simulink model "SF015A_WhlImbRejctn"  (R2013b)
settings: Solver=FixedStepDiscrete  SolverMode=SingleTasking  StartTime=0.0  StopTime=1  FixedStep=0.002  RelTol=1e-3
undefined symbols (not defined in the file): ACTIVBANDMAX_ULS_U32, ADAPVFILMAX_ULS_F32, ADJOUTPMAX_ULS_F32, ARCHGLBPRM_180OVERPI_ULS_F32, ARCHGLBPRM_2MILLISEC_SEC_F32, ARCHGLBPRM_2PI_ULS_F32, ARCHGLBPRM_FLOATZEROTHD_ULS_F32, ARCHGLBPRM_PI_ULS_F32, ARCHGLBPRM_PIOVER180_ULS_F32, ARCHGLBPRM_PIOVER2_ULS_F32, CALMINSPERCOUNT_ULS_F32, Cntr, DURATIONDISABLE_CNT_U16, FILTWHLSPDMAX_MOTRADPERSEC_F32, FRQMIN_ULS_F32, MICROSECTOMILLISEC_ULS_F32, MINSTOMILLISEC_ULS_F32, NINETY_ULS_F32, NODEBSTEP_CNT_U16, NROFDLY_CNT_U08, NtcSts1, NvmGetErrSts1, ONEHALF_ULS_F32, ONEHUNDRED_ULS_F32, ONEOVRTHREE_ULS_F32, ONEOVRTWENTY_ULS_F32, ONETHOUSAND_ULS_F32, PEAKMAX_ULS_F32, PEAKMIN_ULS_F32, PHAADJMAX_ULS_F32, PITIMESSAMPLETIME_ULS_F32, SigQlfr1, STOREDMINSPERCOUNT_ULS_F32, Sts, SysSt1, TWO_ULS_F32, TWOOVRTHREE_ULS_F32, UGRFILMAX_ULS_F32, WhlImbRejctnAdpvFac, WhlImbRejctnAutScaEna, WhlImbRejctnAutScaTar, WhlImbRejctnCurrMgnSlewPerLoop, WhlImbRejctnDcTrendFltRcvryDly, WhlImbRejctnDcTrendFltRcvryNegStep, WhlImbRejctnDcTrendFltRcvryPosStep, WhlImbRejctnDcTrendFltRcvryThd, WhlImbRejctnDcTrendTh2Tq, WhlImbRejctnDcTrendThTq, WhlImbRejctnDcTrendTi2Sec, WhlImbRejctnDcTrendTiSec, WhlImbRejctnEnaSlewPerLoop, WhlImbRejctnFctEna, WhlImbRejctnFltNtc, WhlImbRejctnFrqDiagcAmpThd, WhlImbRejctnFrqDiagcEna, WhlImbRejctnFrqDiagcFltRcvryDly, WhlImbRejctnFrqDiagcFltRcvryNegStep, WhlImbRejctnFrqDiagcFltRcvryPosStep, WhlImbRejctnFrqDiagcFltRcvryThd, WhlImbRejctnFrqDiagcThd ... (+30)
libraries: FixdToFloat x32, simulink x26, NxtrLim x25, Fil x20, NxtrAbslt x9, NxtrMath x7, NxtrMax x6, NxtrMin x4, NxtrNvM x2, FloatToFixd x2, LnrIntrpn x2, NxtrSign x1
(part 9 of 14)

== system SF015A_WhlImbRejctn/WhlImbRejctn/WhlImbRejctnPer2/WIR Low Speed Diagnostics/MaxPersisDiag/If Action Subsystem ==
  In1 : Inport
  Action Port : ActionPort  ActionType=then
  CopyRight2 : Subsystem  Description=|  mask(Copyright Information){none=on}
      | Copyright info block.                                               
      |                                                                     
      | Place copyright information at the top of every subsystem in design.
      mask prompts: none "No parameters"
      mask help: Place copyright information at the top of every subsystem in design.
      mask Display:
      | NxtrConf = 'Nexteer Confidential';
      | 
      | sys = bdroot; %handle for the current model ("system")
      | first = get_param(sys,'Created');
      | if(isempty(first))
      |     first = datestr(now,'yyyy');
      | else
      |     first = first(end-3:end);  %year is last four digits
      | end
      | 
      | last = get_param(sys,'LastModifiedDate');
      | if isempty(last)
      |     last = datestr(now,'yyyy');
      | else
      |     last = last(end-3:end);
      | end
      | 
      | if strcmp(first,last)
      |     fprintf('%s -- Copyright %s Nexteer',NxtrConf,first)
      | else
      |     fprintf('%s -- %s%s- %s Nexteer',NxtrConf,char(169),first,last)
      | end
  Out1 : Outport
  wires:
  In1/1 -> Out1/1

== system SF015A_WhlImbRejctn/WhlImbRejctn/WhlImbRejctnPer2/WIR Low Speed Diagnostics/MaxPersisDiag/Update Persistence Band 3 ==
  NVM Var : Inport
  Condition : Inport  Port=2
  Add : Sum
  Constant3 : Constant  OutDataTypeStr=uint32
  Constant6 : Constant  RequirementInfo={} %GIDa_1d525a57_12aa_4786_b039_fdbfeffc8f33  Value=ACTIVBANDMAX_ULS_U32
  CopyRight2 : Subsystem  Description=|  mask(Copyright Information){none=on}
      | Copyright info block.                                               
      |                                                                     
      | Place copyright information at the top of every subsystem in design.
      mask prompts: none "No parameters"
      mask help: Place copyright information at the top of every subsystem in design.
      mask Display:
      | NxtrConf = 'Nexteer Confidential';
      | 
      | sys = bdroot; %handle for the current model ("system")
      | first = get_param(sys,'Created');
      | first = first(end-3:end);  %year is last four digits
      | 
      | last = get_param(sys,'LastModifiedDate');
      | if isempty(last)
      |     last = datestr(now,'yyyy');
      | else
      |     last = last(end-3:end);
      | end
      | 
      | if strcmp(first,last)
      |     fprintf('%s -- Copyright %s Nexteer',NxtrConf,first)
      | else
      |     fprintf('%s -- %s%s- %s Nexteer',NxtrConf,char(169),first,last)
      | end
  FreqDiagFault1 : Subsystem  RequirementInfo={} %GIDa_be7adfbe_12e3_4d1f_b751_a499999159a7  TreatAsAtomicUnit=on
  If1 : If  RequirementInfo={} %GIDa_0ea92c53_6d11_40e6_981f_8602e62ea0c9  IfExpression=u1
  Logical Operator1 : Logic  AllPortsSameDT=off  OutDataTypeStr=boolean
  Merge1 : Merge
  NoFault1 : Subsystem  RequirementInfo={} %GIDa_03ebdbb3_7e71_4f28_811c_205b7f9dc526  TreatAsAtomicUnit=on
  Relational Operator7 : RelationalOperator  RequirementInfo={} %GIDa_01722b6f_ba93_4b03_83b3_204efa7b0808  Operator=<  OutDataTypeStr=boolean
  UpdateVar : Outport
  wires:
  Logical Operator1/1 -> If1/1
  FreqDiagFault1/1(Output) -> Merge1/1
  NoFault1/1(Output) -> Merge1/2
  If1/1 -> FreqDiagFault1/Action
  If1/2 -> NoFault1/Action
  Constant3/1 -> Add/1
  Add/1 -> FreqDiagFault1/1(Input)
  NVM Var/1 -> [Var]
  Condition/1 -> Logical Operator1/1
  Constant6/1 -> Relational Operator7/2
  Relational Operator7/1 -> Logical Operator1/2
  [Var] -> Relational Operator7/1
  [Var] -> Add/2
  [Var] -> NoFault1/1(Input)
  Merge1/1 -> UpdateVar/1

== system SF015A_WhlImbRejctn/WhlImbRejctn/WhlImbRejctnPer2/WIR Low Speed Diagnostics/MaxPersisDiag/Update Persistence Band1 ==
  NVM Var : Inport
  Condition : Inport  Port=2
  Add : Sum
  Constant3 : Constant  OutDataTypeStr=uint32
  Constant6 : Constant  RequirementInfo={} %GIDa_d3879db0_aaaa_4f96_8253_c1a666713adb  Value=ACTIVBANDMAX_ULS_U32
  CopyRight2 : Subsystem  Description=|  mask(Copyright Information){none=on}
      | Copyright info block.                                               
      |                                                                     
      | Place copyright information at the top of every subsystem in design.
      mask prompts: none "No parameters"
      mask help: Place copyright information at the top of every subsystem in design.
      mask Display:
      | NxtrConf = 'Nexteer Confidential';
      | 
      | sys = bdroot; %handle for the current model ("system")
      | first = get_param(sys,'Created');
      | first = first(end-3:end);  %year is last four digits
      | 
      | last = get_param(sys,'LastModifiedDate');
      | if isempty(last)
      |     last = datestr(now,'yyyy');
      | else
      |     last = last(end-3:end);
      | end
      | 
      | if strcmp(first,last)
      |     fprintf('%s -- Copyright %s Nexteer',NxtrConf,first)
      | else
      |     fprintf('%s -- %s%s- %s Nexteer',NxtrConf,char(169),first,last)
      | end
  FreqDiagFault1 : Subsystem  RequirementInfo={} %GIDa_359f150f_d6cc_4ff0_a268_6ba457e2d369  TreatAsAtomicUnit=on
  If1 : If  RequirementInfo={} %GIDa_06089e48_f5cb_45cb_89f4_21bbb0bce6ae  IfExpression=u1
  Logical Operator1 : Logic  AllPortsSameDT=off  OutDataTypeStr=boolean
  Merge1 : Merge
  NoFault1 : Subsystem  RequirementInfo={} %GIDa_63cd9bcc_abfd_4796_b9a9_88c94dc82f42  TreatAsAtomicUnit=on
  Relational Operator7 : RelationalOperator  RequirementInfo={} %GIDa_95dc9f26_2408_4902_80b2_c9582cdf1274  Operator=<  OutDataTypeStr=boolean
  UpdateVar : Outport
  wires:
  Logical Operator1/1 -> If1/1
  FreqDiagFault1/1(Output) -> Merge1/1
  NoFault1/1(Output) -> Merge1/2
  If1/1 -> FreqDiagFault1/Action
  If1/2 -> NoFault1/Action
  Constant3/1 -> Add/1
  Add/1 -> FreqDiagFault1/1(Input)
  NVM Var/1 -> [Var]
  Condition/1 -> Logical Operator1/1
  Constant6/1 -> Relational Operator7/2
  Relational Operator7/1 -> Logical Operator1/2
  [Var] -> Relational Operator7/1
  [Var] -> NoFault1/1(Input)
  [Var] -> Add/2
  Merge1/1 -> UpdateVar/1

== system SF015A_WhlImbRejctn/WhlImbRejctn/WhlImbRejctnPer2/WIR Low Speed Diagnostics/MaxPersisDiag/Update Persistence Band2 ==
  NVM Var : Inport
  Condition : Inport  Port=2
  Add : Sum
  Constant3 : Constant  OutDataTypeStr=uint32
  Constant6 : Constant  RequirementInfo={} %GIDa_82db90a7_98d3_4902_8915_0b7af750842f  Value=ACTIVBANDMAX_ULS_U32
  CopyRight2 : Subsystem  Description=|  mask(Copyright Information){none=on}
      | Copyright info block.                                               
      |                                                                     
      | Place copyright information at the top of every subsystem in design.
      mask prompts: none "No parameters"
      mask help: Place copyright information at the top of every subsystem in design.
      mask Display:
      | NxtrConf = 'Nexteer Confidential';
      | 
      | sys = bdroot; %handle for the current model ("system")
      | first = get_param(sys,'Created');
      | first = first(end-3:end);  %year is last four digits
      | 
      | last = get_param(sys,'LastModifiedDate');
      | if isempty(last)
      |     last = datestr(now,'yyyy');
      | else
      |     last = last(end-3:end);
      | end
      | 
      | if strcmp(first,last)
      |     fprintf('%s -- Copyright %s Nexteer',NxtrConf,first)
      | else
      |     fprintf('%s -- %s%s- %s Nexteer',NxtrConf,char(169),first,last)
      | end
  FreqDiagFault1 : Subsystem  RequirementInfo={} %GIDa_6ea3fd2e_fad0_4c9e_828f_0553c62f3183  TreatAsAtomicUnit=on
  If1 : If  RequirementInfo={} %GIDa_3d6838fe_19df_4745_9894_1f41b327ce7a  IfExpression=u1
  Logical Operator1 : Logic  AllPortsSameDT=off  OutDataTypeStr=boolean
  Merge1 : Merge
  NoFault1 : Subsystem  RequirementInfo={} %GIDa_4a4caa65_5361_47b0_a88d_ff799b187767  TreatAsAtomicUnit=on
  Relational Operator7 : RelationalOperator  RequirementInfo={} %GIDa_673935b7_bbed_4a45_bb15_19f10e0d5d6b  Operator=<  OutDataTypeStr=boolean
  UpdateVar : Outport
  wires:
  Logical Operator1/1 -> If1/1
  FreqDiagFault1/1(Output) -> Merge1/1
  NoFault1/1(Output) -> Merge1/2
  If1/1 -> FreqDiagFault1/Action
  If1/2 -> NoFault1/Action
  Constant3/1 -> Add/1
  Add/1 -> FreqDiagFault1/1(Input)
  NVM Var/1 -> [Var]
  Condition/1 -> Logical Operator1/1
  [Var] -> Relational Operator7/1
  Constant6/1 -> Relational Operator7/2
  Relational Operator7/1 -> Logical Operator1/2
  [Var] -> Add/2
  [Var] -> NoFault1/1(Input)
  Merge1/1 -> UpdateVar/1

== system SF015A_WhlImbRejctn/WhlImbRejctn/WhlImbRejctnInit1/Check NVM Data/CheckCompPersistence/NoFault/CopyRight2 ==

== system SF015A_WhlImbRejctn/WhlImbRejctn/WhlImbRejctnInit1/Check NVM Data/CheckCompPersistence/Subsystem/CopyRight1 ==

== system SF015A_WhlImbRejctn/WhlImbRejctn/WhlImbRejctnInit1/Check NVM Data/CheckCompPersistence/Subsystem/FreqDiagFault ==
  Input : Inport
  Action Port : ActionPort  ActionType=then
  CopyRight2 : Subsystem  Description=|  mask(Copyright Information){none=on}
      | Copyright info block.                                               
      |                                                                     
      | Place copyright information at the top of every subsystem in design.
      mask prompts: none "No parameters"
      mask help: Place copyright information at the top of every subsystem in design.
      mask Display:
      | NxtrConf = 'Nexteer Confidential';
      | 
      | sys = bdroot; %handle for the current model ("system")
      | first = get_param(sys,'Created');
      | if(isempty(first))
      |     first = datestr(now,'yyyy');
      | else
      |     first = first(end-3:end);  %year is last four digits
      | end
      | 
      | last = get_param(sys,'LastModifiedDate');
      | if isempty(last)
      |     last = datestr(now,'yyyy');
      | else
      |     last = last(end-3:end);
      | end
      | 
      | if strcmp(first,last)
      |     fprintf('%s -- Copyright %s Nexteer',NxtrConf,first)
      | else
      |     fprintf('%s -- %s%s- %s Nexteer',NxtrConf,char(169),first,last)
      | end
  Output : Outport
  wires:
  Input/1 -> Output/1

== system SF015A_WhlImbRejctn/WhlImbRejctn/WhlImbRejctnInit1/Check NVM Data/CheckCompPersistence/Subsystem/NoFault ==
  Input : Inport
  Action Port : ActionPort  ActionType=else
  CopyRight2 : Subsystem  Description=|  mask(Copyright Information){none=on}
      | Copyright info block.                                               
      |                                                                     
      | Place copyright information at the top of every subsystem in design.
      mask prompts: none "No parameters"
      mask help: Place copyright information at the top of every subsystem in design.
      mask Display:
      | NxtrConf = 'Nexteer Confidential';
      | 
      | sys = bdroot; %handle for the current model ("system")
      | first = get_param(sys,'Created');
      | if(isempty(first))
      |     first = datestr(now,'yyyy');
      | else
      |     first = first(end-3:end);  %year is last four digits
      | end
      | 
      | last = get_param(sys,'LastModifiedDate');
      | if isempty(last)
      |     last = datestr(now,'yyyy');
      | else
      |     last = last(end-3:end);
      | end
      | 
      | if strcmp(first,last)
      |     fprintf('%s -- Copyright %s Nexteer',NxtrConf,first)
      | else
      |     fprintf('%s -- %s%s- %s Nexteer',NxtrConf,char(169),first,last)
      | end
  Output : Outport
  wires:
  Input/1 -> Output/1

== system SF015A_WhlImbRejctn/WhlImbRejctn/WhlImbRejctnPer1/Active Rejection Command /Phase Adjust - Floating Point/Calc Filter Coefficients/CalcCoeff ==
  zero : Inport
  pole : Inport  Port=2
  gain : Inport  Port=3
  Add{2,4,6..7} (4 alike) : Sum  Inputs=-+
  Add3 : Sum
  Add5 : Sum
  Constant{1..6} (6 alike) : Constant  OutDataTypeStr=single
  CopyRight2 : Subsystem  Description=|  mask(Copyright Information){none=on}
      | Copyright info block.                                               
      |                                                                     
      | Place copyright information at the top of every subsystem in design.
      mask prompts: none "No parameters"
      mask help: Place copyright information at the top of every subsystem in design.
      mask Display:
      | NxtrConf = 'Nexteer Confidential';
      | 
      | sys = bdroot; %handle for the current model ("system")
      | first = get_param(sys,'Created');
      | if(isempty(first))
      |     first = datestr(now,'yyyy');
      | else
      |     first = first(end-3:end);  %year is last four digits
      | end
      | 
      | last = get_param(sys,'LastModifiedDate');
      | if isempty(last)
      |     last = datestr(now,'yyyy');
      | else
      |     last = last(end-3:end);
      | end
      | 
      | if strcmp(first,last)
      |     fprintf('%s -- Copyright %s Nexteer',NxtrConf,first)
      | else
      |     fprintf('%s -- %s%s- %s Nexteer',NxtrConf,char(169),first,last)
      | end
  Divide1 : Product  Inputs=*/
  Divide3 : Product  Inputs=*/
  Divide4 : Product  Inputs=/*
  Product3 : Product  RndMeth=Zero
  Product4 : Product  Inputs=3
  Unary Minus : UnaryMinus
  Unary Minus1 : UnaryMinus
  z_m : Outport
  p_k : Outport  Port=2
  b_0 : Outport  Port=3
  wires:
  gain/1 -> Product4/3
  pole/1 -> Unary Minus/1
  zero/1 -> Unary Minus1/1
  Product3/1 -> Divide4/1
  Add7/1 -> Product3/1
  Constant6/1 -> Add7/2
  Add6/1 -> Product4/1
  Constant5/1 -> Add6/2
  Divide3/1 -> p_k/1, Add6/1
  Add4/1 -> Divide3/2
  Add5/1 -> Divide3/1
  Constant3/1 -> Add4/2
  Unary Minus/1 -> Add5/2, Add4/1, Product3/2  "s_k"
  Constant4/1 -> Add5/1
  Divide1/1 -> z_m/1, Add7/1
  Add2/1 -> Divide1/2
  Add3/1 -> Divide1/1
  Constant1/1 -> Add2/2
  Unary Minus1/1 -> Product4/2, Add2/1, Add3/2  "sigma_m"
  Constant2/1 -> Add3/1
  Divide4/1 -> b_0/1
  Product4/1 -> Divide4/2

== system SF015A_WhlImbRejctn/WhlImbRejctn/WhlImbRejctnPer1/Active Rejection Command /Phase Adjust - Floating Point/Calc Filter Coefficients/CalcZeroPole ==
  phase : Inport
  freq : Inport  Port=2
  Add3 : Sum  Inputs=+-
  Add4 : Sum
  CheckForZero : Subsystem  RequirementInfo={} %GIDa_f377c22b_44f3_4b44_ade0_a79dfcd1a159  TreatAsAtomicUnit=on
  Constant : Constant  Value=ARCHGLBPRM_PIOVER180_ULS_F32
  Constant1 : Constant  Value=PITIMESSAMPLETIME_ULS_F32
  Constant2 : Constant  OutDataTypeStr=single
  Constant3 : Constant  OutDataTypeStr=single
  CopyRight2 : Subsystem  Description=|  mask(Copyright Information){none=on}
      | Copyright info block.                                               
      |                                                                     
      | Place copyright information at the top of every subsystem in design.
      mask prompts: none "No parameters"
      mask help: Place copyright information at the top of every subsystem in design.
      mask Display:
      | NxtrConf = 'Nexteer Confidential';
      | 
      | sys = bdroot; %handle for the current model ("system")
      | first = get_param(sys,'Created');
      | if(isempty(first))
      |     first = datestr(now,'yyyy');
      | else
      |     first = first(end-3:end);  %year is last four digits
      | end
      | 
      | last = get_param(sys,'LastModifiedDate');
      | if isempty(last)
      |     last = datestr(now,'yyyy');
      | else
      |     last = last(end-3:end);
      | end
      | 
      | if strcmp(first,last)
      |     fprintf('%s -- Copyright %s Nexteer',NxtrConf,first)
      | else
      |     fprintf('%s -- %s%s- %s Nexteer',NxtrConf,char(169),first,last)
      | end
  Divide{,1..3} (4 alike) : Product  Inputs=*/
  Product : Product
  Product1 : Product  RndMeth=Zero
  Product2 : Product
  Sin_f32 : NxtrMath/Sin_f32  SFunctionSpec=single y1 = Sin_f32(single u1)
      settings: AttributesFormatString=%<MaskType>
  Sqrt_f1 : NxtrMath/Sqrt_f32  SFunctionSpec=single y1 = Sqrt_f32(single u1)  ShowSpec=on
      settings: AttributesFormatString=%<MaskType>
  Sqrt_f2 : NxtrMath/Sqrt_f32  SFunctionSpec=single y1 = Sqrt_f32(single u1)  ShowSpec=on
      settings: AttributesFormatString=%<MaskType>
  Sqrt_f3 : NxtrMath/Sqrt_f32  SFunctionSpec=single y1 = Sqrt_f32(single u1)  ShowSpec=on
      settings: AttributesFormatString=%<MaskType>
  gain_at_DC : Constant  OutDataTypeStr=single
  zero : Outport
  pole : Outport  Port=2
  CompGain : Outport  Port=3
  1/Mag at freq : Outport  Port=4
  wires:
  Divide2/1 -> CompGain/1
  [alpha] -> Divide2/2
  gain_at_DC/1 -> Divide2/1
  Product2/1 -> Product1/2, Divide1/1
  Divide1/1 -> pole/1, Divide3/2
  Product1/1 -> zero/1, Divide3/1
  phase/1 -> Product/1
  Sqrt_f2/1 -> Divide1/2
  [alpha] -> Sqrt_f2/1
  Sqrt_f1/1 -> Product1/1
  [alpha] -> Sqrt_f1/1
  Divide/1 -> [alpha]
  Add4/1 -> Divide/2
  Add3/1 -> Divide/1
  Sin_f32/1 -> Add3/2, Add4/1
  Constant3/1 -> Add4/2
  Constant2/1 -> Add3/1
  Product/1 -> Sin_f32/1
  Sqrt_f3/1 -> 1/Mag at freq/1
  Divide3/1 -> Sqrt_f3/1
  Constant/1 -> Product/2
  Constant1/1 -> Product2/2
  freq/1 -> CheckForZero/1(Whl_Freq)
  CheckForZero/1(Freq) -> Product2/1

== system SF015A_WhlImbRejctn/WhlImbRejctn/WhlImbRejctnPer1/Active Rejection Command /Phase Adjust - Floating Point/Calc Filter Coefficients/CopyRight2 ==

== system SF015A_WhlImbRejctn/WhlImbRejctn/WhlImbRejctnPer1/Active Rejection Command /Phase Adjust - Floating Point/Filter 1/CopyRight2 ==

== system SF015A_WhlImbRejctn/WhlImbRejctn/WhlImbRejctnPer1/Active Rejection Command /Phase Adjust - Floating Point/Filter 2/CopyRight2 ==

== system SF015A_WhlImbRejctn/WhlImbRejctn/WhlImbRejctnPer1/Active Rejection Command /Phase Adjust - Floating Point/If Action Subsystem/CopyRight2 ==

== system SF015A_WhlImbRejctn/WhlImbRejctn/WhlImbRejctnPer1/Active Rejection Command /Phase Adjust - Floating Point/If Action Subsystem1/CopyRight2 ==

== system SF015A_WhlImbRejctn/WhlImbRejctn/WhlImbRejctnPer1/Determine Enabled Amt/Calculate Enable1/Check_EnableDisableRange/Check_for_disbale1 ==
  Input : Inport
  Action Port : ActionPort  ActionType=elseif
  CopyRight2 : Subsystem  Description=|  mask(Copyright Information){none=on}
      | Copyright info block.                                               
      |                                                                     
      | Place copyright information at the top of every subsystem in design.
      mask prompts: none "No parameters"
      mask help: Place copyright information at the top of every subsystem in design.
      mask Display:
      | NxtrConf = 'Nexteer Confidential';
      | 
      | sys = bdroot; %handle for the current model ("system")
      | first = get_param(sys,'Created');
      | if(isempty(first))
      |     first = datestr(now,'yyyy');
      | else
      |     first = first(end-3:end);  %year is last four digits
      | end
      | 
      | last = get_param(sys,'LastModifiedDate');
      | if isempty(last)
      |     last = datestr(now,'yyyy');
      | else
      |     last = last(end-3:end);
      | end
      | 
      | if strcmp(first,last)
      |     fprintf('%s -- Copyright %s Nexteer',NxtrConf,first)
      | else
      |     fprintf('%s -- %s%s- %s Nexteer',NxtrConf,char(169),first,last)
      | end
  Output : Outport
  wires:
  Input/1 -> Output/1

== system SF015A_WhlImbRejctn/WhlImbRejctn/WhlImbRejctnPer1/Determine Enabled Amt/Calculate Enable1/Check_EnableDisableRange/Check_for_disbale2 ==
  Input : Inport
  Action Port : ActionPort  ActionType=then
  CopyRight2 : Subsystem  Description=|  mask(Copyright Information){none=on}
      | Copyright info block.                                               
      |                                                                     
      | Place copyright information at the top of every subsystem in design.
      mask prompts: none "No parameters"
      mask help: Place copyright information at the top of every subsystem in design.
      mask Display:
      | NxtrConf = 'Nexteer Confidential';
      | 
      | sys = bdroot; %handle for the current model ("system")
      | first = get_param(sys,'Created');
      | if(isempty(first))
      |     first = datestr(now,'yyyy');
      | else
      |     first = first(end-3:end);  %year is last four digits
      | end
      | 
      | last = get_param(sys,'LastModifiedDate');
      | if isempty(last)
      |     last = datestr(now,'yyyy');
      | else
      |     last = last(end-3:end);
      | end
      | 
      | if strcmp(first,last)
      |     fprintf('%s -- Copyright %s Nexteer',NxtrConf,first)
      | else
      |     fprintf('%s -- %s%s- %s Nexteer',NxtrConf,char(169),first,last)
      | end
  Output : Outport
  wires:
  Input/1 -> Output/1

== system SF015A_WhlImbRejctn/WhlImbRejctn/WhlImbRejctnPer1/Determine Enabled Amt/Calculate Enable1/Check_EnableDisableRange/Check_for_disbale3 ==
  Input : Inport
  Action Port : ActionPort  ActionType=else
  CopyRight2 : Subsystem  Description=|  mask(Copyright Information){none=on}
      | Copyright info block.                                               
      |                                                                     
      | Place copyright information at the top of every subsystem in design.
      mask prompts: none "No parameters"
      mask help: Place copyright information at the top of every subsystem in design.
      mask Display:
      | NxtrConf = 'Nexteer Confidential';
      | 
      | sys = bdroot; %handle for the current model ("system")
      | first = get_param(sys,'Created');
      | if(isempty(first))
      |     first = datestr(now,'yyyy');
      | else
      |     first = first(end-3:end);  %year is last four digits
      | end
      | 
      | last = get_param(sys,'LastModifiedDate');
      | if isempty(last)
      |     last = datestr(now,'yyyy');
      | else
      |     last = last(end-3:end);
      | end
      | 
      | if strcmp(first,last)
      |     fprintf('%s -- Copyright %s Nexteer',NxtrConf,first)
      | else
      |     fprintf('%s -- %s%s- %s Nexteer',NxtrConf,char(169),first,last)
      | end
  Output : Outport
  wires:
  Input/1 -> Output/1

== system SF015A_WhlImbRejctn/WhlImbRejctn/WhlImbRejctnPer1/Determine Enabled Amt/Calculate Enable1/Check_EnableDisableRange/CopyRight2 ==

== system SF015A_WhlImbRejctn/WhlImbRejctn/WhlImbRejctnPer1/Determine Enabled Amt/Calculate Enable1/DistMagL/CopyRight2 ==

== system SF015A_WhlImbRejctn/WhlImbRejctn/WhlImbRejctnPer1/Determine Enabled Amt/Calculate Enable1/DistMagL/PeakLe ==
  Input : Inport
  CurrMag : Inport  Port=2
  Action Port : ActionPort  ActionType=then
  Add : Sum
  Add4 : Sum  Inputs=+-
  Compare To Zero : simulink/Logic and Bit Operations/Compare To Zero  relop=>  OutDataTypeStr=boolean
  Constant1 : Constant  Value=WhlImbRejctnMgnEstimnDeltaSca
  Constant2 : Constant  Value=WhlImbRejctnMgnEstimnLeak
  CopyRight2 : Subsystem  Description=|  mask(Copyright Information){none=on}
      | Copyright info block.                                               
      |                                                                     
      | Place copyright information at the top of every subsystem in design.
      mask prompts: none "No parameters"
      mask help: Place copyright information at the top of every subsystem in design.
      mask Display:
      | NxtrConf = 'Nexteer Confidential';
      | 
      | sys = bdroot; %handle for the current model ("system")
      | first = get_param(sys,'Created');
      | if(isempty(first))
      |     first = datestr(now,'yyyy');
      | else
      |     first = first(end-3:end);  %year is last four digits
      | end
      | 
      | last = get_param(sys,'LastModifiedDate');
      | if isempty(last)
      |     last = datestr(now,'yyyy');
      | else
      |     last = last(end-3:end);
      | end
      | 
      | if strcmp(first,last)
      |     fprintf('%s -- Copyright %s Nexteer',NxtrConf,first)
      | else
      |     fprintf('%s -- %s%s- %s Nexteer',NxtrConf,char(169),first,last)
      | end
  DeltaSca : Subsystem  RequirementInfo={} %GIDa_240c6616_020c_4e97_a7c9_921c156090a8  TreatAsAtomicUnit=on
  If8 : If  RequirementInfo={} %GIDa_c0698fa9_a62d_4e64_a81a_4da5ea4e4d19  IfExpression=u1
  Leak : Subsystem  RequirementInfo={} %GIDa_c4c0cbff_f207_45b7_943c_5cbfb2ef7974  TreatAsAtomicUnit=on
  Merge8 : Merge
  Product1 : Product  RndMeth=Zero
  Product2 : Product  RndMeth=Zero
  Output : Outport
  wires:
  Input/1 -> Add/1, Add4/2, Product1/2
  Compare To Zero/1 -> If8/1
  Constant2/1 -> Product1/1
  Constant1/1 -> Product2/1
  Product2/1 -> Add/2
  CurrMag/1 -> Add4/1
  Add4/1 -> Product2/2, Compare To Zero/1
  If8/1 -> DeltaSca/Action
  If8/2 -> Leak/Action
  Product1/1 -> Leak/1(Input)
  Leak/1(Output) -> Merge8/2
  DeltaSca/1(Output) -> Merge8/1
  Add/1 -> DeltaSca/1(Input)
  Merge8/1 -> Output/1

== system SF015A_WhlImbRejctn/WhlImbRejctn/WhlImbRejctnPer1/Determine Enabled Amt/Calculate Enable1/DistMagL/PrevLe ==
  Input : Inport
  Action Port : ActionPort  ActionType=else
  CopyRight2 : Subsystem  Description=|  mask(Copyright Information){none=on}
      | Copyright info block.                                               
      |                                                                     
      | Place copyright information at the top of every subsystem in design.
      mask prompts: none "No parameters"
      mask help: Place copyright information at the top of every subsystem in design.
      mask Display:
      | NxtrConf = 'Nexteer Confidential';
      | 
      | sys = bdroot; %handle for the current model ("system")
      | first = get_param(sys,'Created');
      | if(isempty(first))
      |     first = datestr(now,'yyyy');
      | else
      |     first = first(end-3:end);  %year is last four digits
      | end
      | 
      | last = get_param(sys,'LastModifiedDate');
      | if isempty(last)
      |     last = datestr(now,'yyyy');
      | else
      |     last = last(end-3:end);
      | end
      | 
      | if strcmp(first,last)
      |     fprintf('%s -- Copyright %s Nexteer',NxtrConf,first)
      | else
      |     fprintf('%s -- %s%s- %s Nexteer',NxtrConf,char(169),first,last)
      | end
  Output : Outport
  wires:
  Input/1 -> Output/1

== system SF015A_WhlImbRejctn/WhlImbRejctn/WhlImbRejctnPer1/Determine Enabled Amt/Calculate Enable1/DistMagR/CopyRight2 ==

== system SF015A_WhlImbRejctn/WhlImbRejctn/WhlImbRejctnPer1/Determine Enabled Amt/Calculate Enable1/DistMagR/PeakRi ==
  Input : Inport
  CurrMag : Inport  Port=2
  Action Port : ActionPort  ActionType=then
  Add3 : Sum
  Add7 : Sum  Inputs=+-
  Compare To Zero1 : simulink/Logic and Bit Operations/Compare To Zero  relop=>  OutDataTypeStr=boolean
  Constant10 : Constant  Value=WhlImbRejctnMgnEstimnLeak
  Constant9 : Constant  Value=WhlImbRejctnMgnEstimnDeltaSca
  CopyRight2 : Subsystem  Description=|  mask(Copyright Information){none=on}
      | Copyright info block.                                               
      |                                                                     
      | Place copyright information at the top of every subsystem in design.
      mask prompts: none "No parameters"
      mask help: Place copyright information at the top of every subsystem in design.
      mask Display:
      | NxtrConf = 'Nexteer Confidential';
      | 
      | sys = bdroot; %handle for the current model ("system")
      | first = get_param(sys,'Created');
      | if(isempty(first))
      |     first = datestr(now,'yyyy');
      | else
      |     first = first(end-3:end);  %year is last four digits
      | end
      | 
      | last = get_param(sys,'LastModifiedDate');
      | if isempty(last)
      |     last = datestr(now,'yyyy');
      | else
      |     last = last(end-3:end);
      | end
      | 
      | if strcmp(first,last)
      |     fprintf('%s -- Copyright %s Nexteer',NxtrConf,first)
      | else
      |     fprintf('%s -- %s%s- %s Nexteer',NxtrConf,char(169),first,last)
      | end
  DeltaSca : Subsystem  RequirementInfo={} %GIDa_f888f5cf_043e_4283_af3d_2c56cdaeddbf  TreatAsAtomicUnit=on
  If8 : If  RequirementInfo={} %GIDa_3248c591_a3b3_4afa_806c_f37d4ef76132  IfExpression=u1
  Leak : Subsystem  RequirementInfo={} %GIDa_f0d5024d_f3e8_4067_92f0_08fd1f0e9ff2  TreatAsAtomicUnit=on
  Merge8 : Merge
  Product4 : Product  RndMeth=Zero
  Product5 : Product  RndMeth=Zero
  Output : Outport
  wires:
  Input/1 -> Add3/1, Add7/2, Product4/2
  Compare To Zero1/1 -> If8/1
  Constant10/1 -> Product4/1
  Constant9/1 -> Product5/1
  Product5/1 -> Add3/2
  CurrMag/1 -> Add7/1
  Add7/1 -> Product5/2, Compare To Zero1/1
  If8/1 -> DeltaSca/Action
  If8/2 -> Leak/Action
  Product4/1 -> Leak/1(Input)
  Leak/1(Output) -> Merge8/2
  DeltaSca/1(Output) -> Merge8/1
  Add3/1 -> DeltaSca/1(Input)
  Merge8/1 -> Output/1

== system SF015A_WhlImbRejctn/WhlImbRejctn/WhlImbRejctnPer1/Determine Enabled Amt/Calculate Enable1/DistMagR/PrevRi ==
  Input : Inport
  Action Port : ActionPort  ActionType=else
  CopyRight2 : Subsystem  Description=|  mask(Copyright Information){none=on}
      | Copyright info block.                                               
      |                                                                     
      | Place copyright information at the top of every subsystem in design.
      mask prompts: none "No parameters"
      mask help: Place copyright information at the top of every subsystem in design.
      mask Display:
      | NxtrConf = 'Nexteer Confidential';
      | 
      | sys = bdroot; %handle for the current model ("system")
      | first = get_param(sys,'Created');
      | if(isempty(first))
      |     first = datestr(now,'yyyy');
      | else
      |     first = first(end-3:end);  %year is last four digits
      | end
      | 
      | last = get_param(sys,'LastModifiedDate');
      | if isempty(last)
      |     last = datestr(now,'yyyy');
      | else
      |     last = last(end-3:end);
      | end
      | 
      | if strcmp(first,last)
      |     fprintf('%s -- Copyright %s Nexteer',NxtrConf,first)
      | else
      |     fprintf('%s -- %s%s- %s Nexteer',NxtrConf,char(169),first,last)
      | end
  Output : Outport
  wires:
  Input/1 -> Output/1

== system SF015A_WhlImbRejctn/WhlImbRejctn/WhlImbRejctnPer1/Determine Enabled Amt/Calculate Enable1/Left_AutoScale/CopyRight2 ==

== system SF015A_WhlImbRejctn/WhlImbRejctn/WhlImbRejctnPer1/Determine Enabled Amt/Calculate Enable1/Left_Enable/CopyRight2 ==

== system SF015A_WhlImbRejctn/WhlImbRejctn/WhlImbRejctnPer1/Determine Enabled Amt/Calculate Enable1/Left_noAutoScale/CopyRight2 ==

== system SF015A_WhlImbRejctn/WhlImbRejctn/WhlImbRejctnPer1/Determine Enabled Amt/Calculate Enable1/Left_noEnable/CopyRight2 ==

== system SF015A_WhlImbRejctn/WhlImbRejctn/WhlImbRejctnPer1/Determine Enabled Amt/Calculate Enable1/Right_AutoScale/CopyRight2 ==

== system SF015A_WhlImbRejctn/WhlImbRejctn/WhlImbRejctnPer1/Determine Enabled Amt/Calculate Enable1/Right_Enable/CopyRight2 ==

== system SF015A_WhlImbRejctn/WhlImbRejctn/WhlImbRejctnPer1/Determine Enabled Amt/Calculate Enable1/Right_noAutoScale/CopyRight2 ==

== system SF015A_WhlImbRejctn/WhlImbRejctn/WhlImbRejctnPer1/Determine Enabled Amt/Calculate Enable1/Right_noEnable/CopyRight2 ==

== system SF015A_WhlImbRejctn/WhlImbRejctn/WhlImbRejctnPer1/Determine Enabled Amt/Calculate Enable1/Use_FreqEst/CopyRight2 ==

== system SF015A_WhlImbRejctn/WhlImbRejctn/WhlImbRejctnPer1/Determine Enabled Amt/Calculate Enable1/Use_Zero/CopyRight2 ==

== system SF015A_WhlImbRejctn/WhlImbRejctn/WhlImbRejctnPer1/Determine Enabled Amt/Calculate Enable1/float 0 output/CopyRight2 ==

== system SF015A_WhlImbRejctn/WhlImbRejctn/WhlImbRejctnPer1/Determine Enabled Amt/Calculate Enable1/float 1 output/CopyRight2 ==

== system SF015A_WhlImbRejctn/WhlImbRejctn/WhlImbRejctnPer1/Determine Enabled Amt/Enable Ramp/ElapsedTime1/CopyRight2 ==

== system SF015A_WhlImbRejctn/WhlImbRejctn/WhlImbRejctnPer1/Determine Enabled Amt/Enable Ramp/ElapsedTime1/If not true elapsed time = 0 ==
  Action Port : ActionPort  ActionType=then
  Constant : Constant  Value=0  OutDataTypeStr=single
  CopyRight2 : Subsystem  Description=|  mask(Copyright Information){none=on}
      | Copyright info block.                                               
      |                                                                     
      | Place copyright information at the top of every subsystem in design.
      mask prompts: none "No parameters"
      mask help: Place copyright information at the top of every subsystem in design.
      mask Display:
      | NxtrConf = 'Nexteer Confidential';
      | 
      | sys = bdroot; %handle for the current model ("system")
      | first = get_param(sys,'Created');
      | if(isempty(first))
      |     first = datestr(now,'yyyy');
      | else
      |     first = first(end-3:end);  %year is last four digits
      | end
      | 
      | last = get_param(sys,'LastModifiedDate');
      | if isempty(last)
      |     last = datestr(now,'yyyy');
      | else
      |     last = last(end-3:end);
      | end
      | 
      | if strcmp(first,last)
      |     fprintf('%s -- Copyright %s Nexteer',NxtrConf,first)
      | else
      |     fprintf('%s -- %s%s- %s Nexteer',NxtrConf,char(169),first,last)
      | end
  SpanTi : Outport
  wires:
  Constant/1 -> SpanTi/1

== system SF015A_WhlImbRejctn/WhlImbRejctn/WhlImbRejctnPer1/Determine Enabled Amt/Enable Ramp/ElapsedTime1/If true and last step is true calculate elapsed time  ==
  Action Port : ActionPort  ActionType=else
  Constant1 : Constant  Value=MICROSECTOMILLISEC_ULS_F32
  CopyRight2 : Subsystem  Description=|  mask(Copyright Information){none=on}
      | Copyright info block.                                               
      |                                                                     
      | Place copyright information at the top of every subsystem in design.
      mask prompts: none "No parameters"
      mask help: Place copyright information at the top of every subsystem in design.
      mask Display:
      | NxtrConf = 'Nexteer Confidential';
      | 
      | sys = bdroot; %handle for the current model ("system")
      | first = get_param(sys,'Created');
      | if(isempty(first))
      |     first = datestr(now,'yyyy');
      | else
      |     first = first(end-3:end);  %year is last four digits
      | end
      | 
      | last = get_param(sys,'LastModifiedDate');
      | if isempty(last)
      |     last = datestr(now,'yyyy');
      | else
      |     last = last(end-3:end);
      | end
      | 
      | if strcmp(first,last)
      |     fprintf('%s -- Copyright %s Nexteer',NxtrConf,first)
      | else
      |     fprintf('%s -- %s%s- %s Nexteer',NxtrConf,char(169),first,last)
      | end
  Data Store Read : DataStoreRead  DataStoreName=SlowSpdDiagcRefTiEnaLrngTmr
  Divide : Product  Inputs=**
  FixdToFloat_f32_u32 : FixdToFloat/FixdToFloat_f32_u32  Param1=0
  GetTiSpan100MicroSec32bit : Subsystem
  SpanTi : Outport
  wires:
  Divide/1 -> SpanTi/1
  GetTiSpan100MicroSec32bit/1(TiSpan) -> FixdToFloat_f32_u32/1
  Data Store Read/1 -> GetTiSpan100MicroSec32bit/1(RefTmr)
  FixdToFloat_f32_u32/1 -> Divide/1
  Constant1/1 -> Divide/2

== system SF015A_WhlImbRejctn/WhlImbRejctn/WhlImbRejctnPer1/Determine Enabled Amt/Enable Ramp/ElapsedTime1/If true and last step not true elapsed time = 0 get reference time  ==
  Action Port : ActionPort  ActionType=elseif
  Constant : Constant  Value=0  OutDataTypeStr=single
  CopyRight2 : Subsystem  Description=|  mask(Copyright Information){none=on}
      | Copyright info block.                                               
      |                                                                     
      | Place copyright information at the top of every subsystem in design.
      mask prompts: none "No parameters"
      mask help: Place copyright information at the top of every subsystem in design.
      mask Display:
      | NxtrConf = 'Nexteer Confidential';
      | 
      | sys = bdroot; %handle for the current model ("system")
      | first = get_param(sys,'Created');
      | if(isempty(first))
      |     first = datestr(now,'yyyy');
      | else
      |     first = first(end-3:end);  %year is last four digits
      | end
      | 
      | last = get_param(sys,'LastModifiedDate');
      | if isempty(last)
      |     last = datestr(now,'yyyy');
      | else
      |     last = last(end-3:end);
      | end
      | 
      | if strcmp(first,last)
      |     fprintf('%s -- Copyright %s Nexteer',NxtrConf,first)
      | else
      |     fprintf('%s -- %s%s- %s Nexteer',NxtrConf,char(169),first,last)
      | end
  Data Store Write : DataStoreWrite  DataStoreName=SlowSpdDiagcRefTiEnaLrngTmr
  GetRefTmr100MicroSec32bit : Subsystem
  "SpanTi " : Outport
  wires:
  Constant/1 -> "SpanTi "/1
  GetRefTmr100MicroSec32bit/1(RefTmr) -> Data Store Write/1

== system SF015A_WhlImbRejctn/WhlImbRejctn/WhlImbRejctnPer1/Determine Enabled Amt/Enable Ramp/NoFaultOper/CopyRight2 ==

== system SF015A_WhlImbRejctn/WhlImbRejctn/WhlImbRejctnPer1/Determine Enabled Amt/Enable Ramp/Reset WIR /CopyRight2 ==

== system SF015A_WhlImbRejctn/WhlImbRejctn/WhlImbRejctnPer1/Determine Enabled Amt/Enable Ramp/Right_active1/CopyRight2 ==

== system SF015A_WhlImbRejctn/WhlImbRejctn/WhlImbRejctnPer1/Determine Enabled Amt/Enable Ramp/Right_noactive1/CopyRight2 ==

== system SF015A_WhlImbRejctn/WhlImbRejctn/WhlImbRejctnPer1/Determine Enabled Amt/Enable Ramp/SlowSpeedDiagcCalc/CopyRight2 ==

== system SF015A_WhlImbRejctn/WhlImbRejctn/WhlImbRejctnPer1/WIR Diagnostics/DcTrendDiag/DCTrendFault/CopyRight2 ==

== system SF015A_WhlImbRejctn/WhlImbRejctn/WhlImbRejctnPer1/WIR Diagnostics/DcTrendDiag/ElapsedTime1/CopyRight2 ==

== system SF015A_WhlImbRejctn/WhlImbRejctn/WhlImbRejctnPer1/WIR Diagnostics/DcTrendDiag/ElapsedTime1/If not true elapsed time = 0 ==
  Action Port : ActionPort  ActionType=then
  Constant : Constant  Value=0  OutDataTypeStr=single
  CopyRight2 : Subsystem  Description=|  mask(Copyright Information){none=on}
      | Copyright info block.                                               
      |                                                                     
      | Place copyright information at the top of every subsystem in design.
      mask prompts: none "No parameters"
      mask help: Place copyright information at the top of every subsystem in design.
      mask Display:
      | NxtrConf = 'Nexteer Confidential';
      | 
      | sys = bdroot; %handle for the current model ("system")
      | first = get_param(sys,'Created');
      | if(isempty(first))
      |     first = datestr(now,'yyyy');
      | else
      |     first = first(end-3:end);  %year is last four digits
      | end
      | 
      | last = get_param(sys,'LastModifiedDate');
      | if isempty(last)
      |     last = datestr(now,'yyyy');
      | else
      |     last = last(end-3:end);
      | end
      | 
      | if strcmp(first,last)
      |     fprintf('%s -- Copyright %s Nexteer',NxtrConf,first)
      | else
      |     fprintf('%s -- %s%s- %s Nexteer',NxtrConf,char(169),first,last)
      | end
  SpanTi : Outport
  wires:
  Constant/1 -> SpanTi/1

== system SF015A_WhlImbRejctn/WhlImbRejctn/WhlImbRejctnPer1/WIR Diagnostics/DcTrendDiag/ElapsedTime1/If true and last step is true calculate elapsed time  ==
  Action Port : ActionPort  ActionType=else
  Constant1 : Constant  Value=MICROSECTOMILLISEC_ULS_F32
  CopyRight2 : Subsystem  Description=|  mask(Copyright Information){none=on}
      | Copyright info block.                                               
      |                                                                     
      | Place copyright information at the top of every subsystem in design.
      mask prompts: none "No parameters"
      mask help: Place copyright information at the top of every subsystem in design.
      mask Display:
      | NxtrConf = 'Nexteer Confidential';
      | 
      | sys = bdroot; %handle for the current model ("system")
      | first = get_param(sys,'Created');
      | if(isempty(first))
      |     first = datestr(now,'yyyy');
      | else
      |     first = first(end-3:end);  %year is last four digits
      | end
      | 
      | last = get_param(sys,'LastModifiedDate');
      | if isempty(last)
      |     last = datestr(now,'yyyy');
      | else
      |     last = last(end-3:end);
      | end
      | 
      | if strcmp(first,last)
      |     fprintf('%s -- Copyright %s Nexteer',NxtrConf,first)
      | else
      |     fprintf('%s -- %s%s- %s Nexteer',NxtrConf,char(169),first,last)
      | end
  Data Store Read : DataStoreRead  DataStoreName=DcTrendRefTiEnaLrngTmr1
  Divide : Product  Inputs=**
  FixdToFloat_f32_u32 : FixdToFloat/FixdToFloat_f32_u32  Param1=0
  GetTiSpan100MicroSec 32bit : Subsystem
  SpanTi : Outport
  wires:
  Constant1/1 -> Divide/2
  Divide/1 -> SpanTi/1
  GetTiSpan100MicroSec 32bit/1(TiSpan) -> FixdToFloat_f32_u32/1
  Data Store Read/1 -> GetTiSpan100MicroSec 32bit/1(RefTmr)
  FixdToFloat_f32_u32/1 -> Divide/1

== system SF015A_WhlImbRejctn/WhlImbRejctn/WhlImbRejctnPer1/WIR Diagnostics/DcTrendDiag/ElapsedTime1/If true and last step not true elapsed time = 0 get reference time  ==
  Action Port : ActionPort  ActionType=elseif
  Constant : Constant  Value=0  OutDataTypeStr=single
  CopyRight2 : Subsystem  Description=|  mask(Copyright Information){none=on}
      | Copyright info block.                                               
      |                                                                     
      | Place copyright information at the top of every subsystem in design.
      mask prompts: none "No parameters"
      mask help: Place copyright information at the top of every subsystem in design.
      mask Display:
      | NxtrConf = 'Nexteer Confidential';
      | 
      | sys = bdroot; %handle for the current model ("system")
      | first = get_param(sys,'Created');
      | if(isempty(first))
      |     first = datestr(now,'yyyy');
      | else
      |     first = first(end-3:end);  %year is last four digits
      | end
      | 
      | last = get_param(sys,'LastModifiedDate');
      | if isempty(last)
      |     last = datestr(now,'yyyy');
      | else
      |     last = last(end-3:end);
      | end
      | 
      | if strcmp(first,last)
      |     fprintf('%s -- Copyright %s Nexteer',NxtrConf,first)
      | else
      |     fprintf('%s -- %s%s- %s Nexteer',NxtrConf,char(169),first,last)
      | end
  Data Store Write : DataStoreWrite  DataStoreName=DcTrendRefTiEnaLrngTmr1
  GetRefTmr100MicroSec32bit : Subsystem
  "SpanTi " : Outport
  wires:
  Constant/1 -> "SpanTi "/1
  GetRefTmr100MicroSec32bit/1(RefTmr) -> Data Store Write/1

== system SF015A_WhlImbRejctn/WhlImbRejctn/WhlImbRejctnPer1/WIR Diagnostics/DcTrendDiag/ElapsedTime2/CopyRight2 ==

== system SF015A_WhlImbRejctn/WhlImbRejctn/WhlImbRejctnPer1/WIR Diagnostics/DcTrendDiag/ElapsedTime2/If not true elapsed time = 0 ==
  Action Port : ActionPort  ActionType=then
  Constant : Constant  Value=0  OutDataTypeStr=single
  CopyRight2 : Subsystem  Description=|  mask(Copyright Information){none=on}
      | Copyright info block.                                               
      |                                                                     
      | Place copyright information at the top of every subsystem in design.
      mask prompts: none "No parameters"
      mask help: Place copyright information at the top of every subsystem in design.
      mask Display:
      | NxtrConf = 'Nexteer Confidential';
      | 
      | sys = bdroot; %handle for the current model ("system")
      | first = get_param(sys,'Created');
      | if(isempty(first))
      |     first = datestr(now,'yyyy');
      | else
      |     first = first(end-3:end);  %year is last four digits
      | end
      | 
      | last = get_param(sys,'LastModifiedDate');
      | if isempty(last)
      |     last = datestr(now,'yyyy');
      | else
      |     last = last(end-3:end);
      | end
      | 
      | if strcmp(first,last)
      |     fprintf('%s -- Copyright %s Nexteer',NxtrConf,first)
      | else
      |     fprintf('%s -- %s%s- %s Nexteer',NxtrConf,char(169),first,last)
      | end
  SpanTi : Outport
  wires:
  Constant/1 -> SpanTi/1

== system SF015A_WhlImbRejctn/WhlImbRejctn/WhlImbRejctnPer1/WIR Diagnostics/DcTrendDiag/ElapsedTime2/If true and last step is true calculate elapsed time  ==
  Action Port : ActionPort  ActionType=else
  Constant1 : Constant  Value=MICROSECTOMILLISEC_ULS_F32
  CopyRight2 : Subsystem  Description=|  mask(Copyright Information){none=on}
      | Copyright info block.                                               
      |                                                                     
      | Place copyright information at the top of every subsystem in design.
      mask prompts: none "No parameters"
      mask help: Place copyright information at the top of every subsystem in design.
      mask Display:
      | NxtrConf = 'Nexteer Confidential';
      | 
      | sys = bdroot; %handle for the current model ("system")
      | first = get_param(sys,'Created');
      | if(isempty(first))
      |     first = datestr(now,'yyyy');
      | else
      |     first = first(end-3:end);  %year is last four digits
      | end
      | 
      | last = get_param(sys,'LastModifiedDate');
      | if isempty(last)
      |     last = datestr(now,'yyyy');
      | else
      |     last = last(end-3:end);
      | end
      | 
      | if strcmp(first,last)
      |     fprintf('%s -- Copyright %s Nexteer',NxtrConf,first)
      | else
      |     fprintf('%s -- %s%s- %s Nexteer',NxtrConf,char(169),first,last)
      | end
  Data Store Read : DataStoreRead  DataStoreName=DcTrendRefTiEnaLrngTmr2
  Divide : Product  Inputs=**
  FixdToFloat_f32_u32 : FixdToFloat/FixdToFloat_f32_u32  Param1=0
  GetTiSpan100MicroSec32bit : Subsystem
  SpanTi : Outport
  wires:
  Constant1/1 -> Divide/2
  Divide/1 -> SpanTi/1
  GetTiSpan100MicroSec32bit/1(TiSpan) -> FixdToFloat_f32_u32/1
  Data Store Read/1 -> GetTiSpan100MicroSec32bit/1(RefTmr)
  FixdToFloat_f32_u32/1 -> Divide/1

== system SF015A_WhlImbRejctn/WhlImbRejctn/WhlImbRejctnPer1/WIR Diagnostics/DcTrendDiag/ElapsedTime2/If true and last step not true elapsed time = 0 get reference time  ==
  Action Port : ActionPort  ActionType=elseif
  Constant : Constant  Value=0  OutDataTypeStr=single
  CopyRight2 : Subsystem  Description=|  mask(Copyright Information){none=on}
      | Copyright info block.                                               
      |                                                                     
      | Place copyright information at the top of every subsystem in design.
      mask prompts: none "No parameters"
      mask help: Place copyright information at the top of every subsystem in design.
      mask Display:
      | NxtrConf = 'Nexteer Confidential';
      | 
      | sys = bdroot; %handle for the current model ("system")
      | first = get_param(sys,'Created');
      | if(isempty(first))
      |     first = datestr(now,'yyyy');
      | else
      |     first = first(end-3:end);  %year is last four digits
      | end
      | 
      | last = get_param(sys,'LastModifiedDate');
      | if isempty(last)
      |     last = datestr(now,'yyyy');
      | else
      |     last = last(end-3:end);
      | end
      | 
      | if strcmp(first,last)
      |     fprintf('%s -- Copyright %s Nexteer',NxtrConf,first)
      | else
      |     fprintf('%s -- %s%s- %s Nexteer',NxtrConf,char(169),first,last)
      | end
  Data Store Write : DataStoreWrite  DataStoreName=DcTrendRefTiEnaLrngTmr2
  GetRefTmr100MicroSec32bit : Subsystem
  "SpanTi " : Outport
  wires:
  Constant/1 -> "SpanTi "/1
  GetRefTmr100MicroSec32bit/1(RefTmr) -> Data Store Write/1

== system SF015A_WhlImbRejctn/WhlImbRejctn/WhlImbRejctnPer1/WIR Diagnostics/DcTrendDiag/Fault_RcvryPath/CopyRight2 ==
